simulink model "SS_passive_damping"  (R2018b)
settings: Solver=ode4  StartTime=0.0  StopTime=300  FixedStep=0.02  RelTol=1e-3
values from neighbouring files (symbols this model uses):
  L = -[G_01 G_02 G_03 G_04]'    [SSModel_calc.m]
  SS_full = ss(A_wec,B_wec,C_wec,D_wec)    [SSModel_calc.m]
settings Model: Creator=user  LastModifiedBy=user

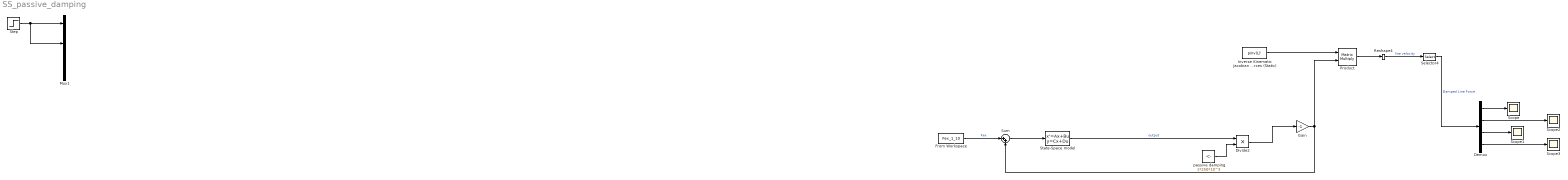
== system SS_passive_damping ==
  Demux : Demux
  Divide2 : Product  Inputs=**
  From Workspace : FromWorkspace  VariableName=Fex_1_10  SampleTime=0
  Gain : Gain  Gain=-1
  Inverse Kinematic Jacobian Go from 6 Cart forces to 4 line forces (Static) : Constant  Value=pinv(L)'
  Mux1 : Mux  Inputs=6
  Product : Product  Multiplication=Matrix(*)
  Reshape4 : Reshape  OutputDimensionality=Column vector (2-D)
  Scope{,1..3} (4 alike) : Scope
  Selector4 : Selector  InputPortWidth=4  IndexOptions=Index vector (dialog)  Indices=[1:4]  OutputSizes=1
  State-Space model : StateSpace  A=SS_full.A  B=SS_full.B  C=SS_full.C  D=SS_full.D  InitialCondition=0
  Step : Step  Time=20  SampleTime=0
  Sum : Sum  Inputs=|++
  passive damping : Constant  Value=1*250*10^3
  wires:
  From Workspace/1 -> Sum/1  "Fex"
  Step/1 -> Mux1/3, Mux1/1
  Product/1 -> Reshape4/1
  Selector4/1 -> Demux/1  "Damped Line Force"
  passive damping/1 -> Divide2/2
  State-Space model/1 -> Divide2/1  "output"
  Inverse Kinematic Jacobian Go from 6 Cart forces to 4 line forces (Static)/1 -> Product/1
  Reshape4/1 -> Selector4/1  "line velocity"
  Gain/1 -> Sum/2, Product/2
  Demux/1 -> Scope/1
  Demux/3 -> Scope1/1
  Demux/2 -> Scope2/1
  Demux/4 -> Scope3/1
  Divide2/1 -> Gain/1
  Sum/1 -> State-Space model/1
